simulink model "tetherForce"  (R2018b)
settings: Solver=VariableStepAuto  StartTime=0.0  StopTime=tsim  RelTol=1e-3
undefined symbols (not defined in the file or in its folder): lz, tetherk, xy
libraries: vrlib x3
settings Model: Creator=Erin B  LastModifiedBy=Erin B

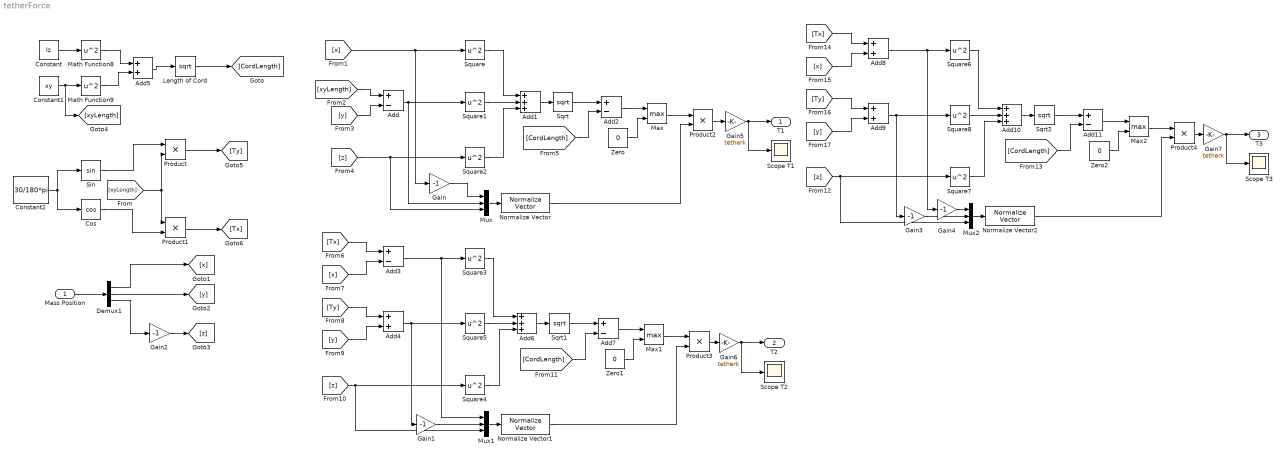
== system tetherForce ==
  Mass Position : Inport
  Add{,2..3,7,11} (5 alike) : Sum  Inputs=+-
  Add1 : Sum  Inputs=+++
  Add10 : Sum  Inputs=+++
  Add{4..5,8..9} (4 alike) : Sum
  Add6 : Sum  Inputs=+++
  Constant : Constant  Value=lz
  Constant1 : Constant  Value=xy
  Constant2 : Constant  Value=30/180*pi
  Cos : Trigonometry  Operator=cos
  Demux1 : Demux  Outputs=3
  Gain{,1..4} (5 alike) : Gain  Gain=-1
  Gain5 : Gain  Gain=tetherk
  Gain6 : Gain  Gain=tetherk
  Gain7 : Gain  Gain=tetherk
  Length of Cord : Sqrt  SaturateOnIntegerOverflow=on
  Math Function8 : Math  Operator=square  SaturateOnIntegerOverflow=on
  Math Function9 : Math  Operator=square  SaturateOnIntegerOverflow=on
  Max : MinMax  Function=max  Inputs=2
  Max1 : MinMax  Function=max  Inputs=2
  Max2 : MinMax  Function=max  Inputs=2
  Mux : Mux  Inputs=3
  Mux1 : Mux  Inputs=3
  Mux2 : Mux  Inputs=3
  Normalize Vector : vrlib/Utilities/Normalize Vector  maxzero=0
      settings: SourceProductName=Simulink 3D Animation  SourceProductBaseCode=VR
  Normalize Vector1 : vrlib/Utilities/Normalize Vector  maxzero=0
      settings: SourceProductName=Simulink 3D Animation  SourceProductBaseCode=VR
  Normalize Vector2 : vrlib/Utilities/Normalize Vector  maxzero=0
      settings: SourceProductName=Simulink 3D Animation  SourceProductBaseCode=VR
  Product{,1..4} (5 alike) : Product
  Scope T1 : Scope
  Scope T2 : Scope
  Scope T3 : Scope
  Sin : Trigonometry
  Sqrt : Sqrt  SaturateOnIntegerOverflow=on
  Sqrt1 : Sqrt  SaturateOnIntegerOverflow=on
  Sqrt2 : Sqrt  SaturateOnIntegerOverflow=on
  Square{,1..8} (9 alike) : Math  Operator=square  SaturateOnIntegerOverflow=on
  Zero : Constant  Value=0  OutDataTypeStr=Inherit: Inherit via back propagation
  Zero1 : Constant  Value=0  OutDataTypeStr=Inherit: Inherit via back propagation
  Zero2 : Constant  Value=0  OutDataTypeStr=Inherit: Inherit via back propagation
  T1 : Outport
  T2 : Outport  Port=2
  T3 : Outport  Port=3
  wires:
  Constant2/1 -> Sin/1, Cos/1
  Sin/1 -> Product/1
  Cos/1 -> Product1/2
  Math Function9/1 -> Add5/2
  Constant1/1 -> [xyLength], Math Function9/1
  Math Function8/1 -> Add5/1
  Add5/1 -> Length of Cord/1
  Length of Cord/1 -> [CordLength]
  Constant/1 -> Math Function8/1
  Mass Position/1 -> Demux1/1
  Gain2/1 -> [z]
  Demux1/2 -> [y]
  Demux1/3 -> Gain2/1
  Demux1/1 -> [x]
  [xyLength] -> Product1/1, Product/2
  Product/1 -> [Ty]
  Product1/1 -> [Tx]
  [y] -> Add/2
  [x] -> Gain/1, Square/1
  [z] -> Mux/3, Square2/1
  Add/1 -> Mux/2, Square1/1
  Square1/1 -> Add1/2
  Square/1 -> Add1/1
  Square2/1 -> Add1/3
  Mux/1 -> Normalize Vector/1
  Gain/1 -> Mux/1
  Add1/1 -> Sqrt/1
  Sqrt/1 -> Add2/1
  [CordLength] -> Add2/2
  Add2/1 -> Max/1
  Zero/1 -> Max/2
  Max/1 -> Product2/1
  Normalize Vector/1 -> Product2/2
  [Tx] -> Add3/1
  [x] -> Add3/2
  [Ty] -> Add4/1
  [y] -> Add4/2
  [z] -> Mux1/3, Square4/1
  Add4/1 -> Gain1/1, Square5/1
  Add3/1 -> Square3/1, Mux1/1
  [CordLength] -> Add7/2
  Add7/1 -> Max1/1
  Square4/1 -> Add6/3
  Normalize Vector1/1 -> Product3/2
  Add6/1 -> Sqrt1/1
  Square3/1 -> Add6/1
  Square5/1 -> Add6/2
  Max1/1 -> Product3/1
  Sqrt1/1 -> Add7/1
  Zero1/1 -> Max1/2
  Mux1/1 -> Normalize Vector1/1
  Gain1/1 -> Mux1/2
  [x] -> Add8/2
  Square6/1 -> Add10/1
  Square7/1 -> Add10/3
  Gain3/1 -> Mux2/2
  [y] -> Add9/2
  Add8/1 -> Gain4/1, Square6/1
  Add9/1 -> Gain3/1, Square8/1
  Normalize Vector2/1 -> Product4/2
  Square8/1 -> Add10/2
  [Tx] -> Add8/1
  Sqrt2/1 -> Add11/1
  Zero2/1 -> Max2/2
  [z] -> Mux2/3, Square7/1
  Max2/1 -> Product4/1
  [Ty] -> Add9/1
  Add10/1 -> Sqrt2/1
  Add11/1 -> Max2/1
  [CordLength] -> Add11/2
  Mux2/1 -> Normalize Vector2/1
  Gain4/1 -> Mux2/1
  Product2/1 -> Gain5/1
  Gain5/1 -> Scope T1/1, T1/1
  Product3/1 -> Gain6/1
  Gain6/1 -> Scope T2/1, T2/1
  Product4/1 -> Gain7/1
  Gain7/1 -> Scope T3/1, T3/1
  [xyLength] -> Add/1
